simulink model "ProcessNetworkSimulation"  (R2015b)
settings: Solver=VariableStepAuto  StartTime=0.0  StopTime=1000.0  RelTol=1e-3
libraries: simulink x1, simeventslib x1
(part 20 of 21)

== system ProcessNetworkSimulation/Process_73/Process ==
  OUTQueue : FIFOQueue  Capacity=inf
  ProcessQueue : FIFOQueue  Capacity=Inf  StatAverageWait=on  StatAverageQueueLength=on
      settings: OutputPortMap=o2,o3
  ProcessServer : NServer  NumberOfServers=14  ServiceTimeFrom=Signal port t  StatNumberDeparted=on  StatUtilization=on
      settings: OutputPortMap=o0,o5
  ProcessTime : EventBasedRandomNumber  meanExp=0.05  minUnif=1  meanNorm=2  stdNorm=0.2  Seed=56201
  Routing : EventBasedRandomNumber  Distribution=Arbitrary discrete  valueVecDisc=[0,1,2,3,4,5,6,7,8,9,10,11,12,13,14,15,16,17,18,19,20,21,22,23,24,25,26,27,28,29,30,31,32,33,34,35,36,37,38,39,40,41,42,43,44]  probVecDisc=[0,0.032,0.0036,0.0071,0.0285,0.032,0.0071,0.032,0.0214,0.0249,0.0214,0.032,0.0036,0.032,0.0285,0.0249,0.0249,0.0249,0.0214,0.032,0.032,0.032,0.0249,0.0285,0.0249,0.0178,0.0214,0.032,0.032,0.0071,0.0071,0.032,0.0036,0.0356,0.0214,0.032,0.0249,0.0249,0.032,0.0107,0.0071,0.0214,0.0249,0.0285,0.0071]  Seed=59418
  read_ProcessTimer : ReadTimer  TimerTag=T_Process_73  StatAverageTimeElapsed=on
      settings: OutputPortMap=o3
  setRouting : SetAttribute  AttributeName=outputFlowNode  AttributeFrom=Signal port  EvaluatedAttributeValue={ []}
  start_ProcessTimer : StartTimer  TimerTag=T_Process_73  TimerStartedOption=Restart
  IN_Job : PMIOPort  Port=1  Side=Left
  OUT_Job : PMIOPort  Port=2  Side=Right
  wires:
  Routing/1 -> setRouting/1
  ProcessTime/1 -> ProcessServer/1
  connections:
  setRouting/LConn1 -- OUTQueue/RConn1
  IN_Job/RConn1 -- start_ProcessTimer/LConn1
  ProcessServer/RConn1 -- read_ProcessTimer/LConn1
  start_ProcessTimer/RConn1 -- ProcessQueue/LConn1
  ProcessQueue/RConn1 -- ProcessServer/LConn1
  read_ProcessTimer/RConn1 -- OUTQueue/LConn1
  OUT_Job/RConn1 -- setRouting/RConn1

== system ProcessNetworkSimulation/Process_74/Process ==
  OUTQueue : FIFOQueue  Capacity=inf
  ProcessQueue : FIFOQueue  Capacity=Inf  StatAverageWait=on  StatAverageQueueLength=on
      settings: OutputPortMap=o2,o3
  ProcessServer : NServer  NumberOfServers=8  ServiceTimeFrom=Signal port t  StatNumberDeparted=on  StatUtilization=on
      settings: OutputPortMap=o0,o5
  ProcessTime : EventBasedRandomNumber  meanExp=0.05  minUnif=1  meanNorm=2  stdNorm=0.2  Seed=62635
  Routing : EventBasedRandomNumber  Distribution=Arbitrary discrete  valueVecDisc=[0,1,2,3,4,5,6,7,8,9,10,11,12,13,14,15,16,17,18,19,20,21,22,23,24,25,26,27,28,29,30,31,32,33,34,35]  probVecDisc=[0,0.0511,0.0146,0.0146,0.0657,0.0219,0.0438,0.0365,0.0511,0.0365,0.0146,0.0146,0.0146,0.0657,0.0365,0.0146,0.0073,0.0146,0.0729,0.0365,0.0219,0.0219,0.0219,0.0146,0.0073,0.0146,0.0511,0.0365,0.0219,0.0146,0.0146,0.0073,0.0146,0.0438,0.0657,0]  Seed=316
  read_ProcessTimer : ReadTimer  TimerTag=T_Process_74  StatAverageTimeElapsed=on
      settings: OutputPortMap=o3
  setRouting : SetAttribute  AttributeName=outputFlowNode  AttributeFrom=Signal port  EvaluatedAttributeValue={ []}
  start_ProcessTimer : StartTimer  TimerTag=T_Process_74  TimerStartedOption=Restart
  IN_Job : PMIOPort  Port=1  Side=Left
  OUT_Job : PMIOPort  Port=2  Side=Right
  wires:
  Routing/1 -> setRouting/1
  ProcessTime/1 -> ProcessServer/1
  connections:
  setRouting/LConn1 -- OUTQueue/RConn1
  IN_Job/RConn1 -- start_ProcessTimer/LConn1
  ProcessServer/RConn1 -- read_ProcessTimer/LConn1
  start_ProcessTimer/RConn1 -- ProcessQueue/LConn1
  ProcessQueue/RConn1 -- ProcessServer/LConn1
  read_ProcessTimer/RConn1 -- OUTQueue/LConn1
  OUT_Job/RConn1 -- setRouting/RConn1

== system ProcessNetworkSimulation/Process_75/Process ==
  OUTQueue : FIFOQueue  Capacity=inf
  ProcessQueue : FIFOQueue  Capacity=Inf  StatAverageWait=on  StatAverageQueueLength=on
      settings: OutputPortMap=o2,o3
  ProcessServer : NServer  NumberOfServers=13  ServiceTimeFrom=Signal port t  StatNumberDeparted=on  StatUtilization=on
      settings: OutputPortMap=o0,o5
  ProcessTime : EventBasedRandomNumber  meanExp=0.05  minUnif=1  meanNorm=2  stdNorm=0.2  Seed=3533
  Routing : EventBasedRandomNumber  Distribution=Arbitrary discrete  valueVecDisc=[0,1,2,3,4,5,6,7,8,9,10,11,12,13,14,15,16,17,18,19,20,21,22,23,24,25,26,27,28,29,30,31,32,33,34,35,36,37,38,39,40,41,42,43,44,45,46,47,48,49,50]  probVecDisc=[0,0.0081,0.0242,0.0242,0.0242,0.004,0.0121,0.0363,0.0121,0.0081,0.0081,0.0363,0.0282,0.0397,0.0363,0.0081,0.0282,0.0081,0.0081,0.0323,0.0202,0.0363,0.0081,0.0202,0.0282,0.0081,0.0202,0.0081,0.004,0.0363,0.0121,0.0081,0.0242,0.0282,0.0363,0.0202,0.0242,0.0081,0.0282,0.0081,0.0363,0.0081,0.0282,0.0081,0.0242,0.0121,0.0242,0.0081,0.0403,0.0363,0]  Seed=6750
  read_ProcessTimer : ReadTimer  TimerTag=T_Process_75  StatAverageTimeElapsed=on
      settings: OutputPortMap=o3
  setRouting : SetAttribute  AttributeName=outputFlowNode  AttributeFrom=Signal port  EvaluatedAttributeValue={ []}
  start_ProcessTimer : StartTimer  TimerTag=T_Process_75  TimerStartedOption=Restart
  IN_Job : PMIOPort  Port=1  Side=Left
  OUT_Job : PMIOPort  Port=2  Side=Right
  wires:
  Routing/1 -> setRouting/1
  ProcessTime/1 -> ProcessServer/1
  connections:
  setRouting/LConn1 -- OUTQueue/RConn1
  IN_Job/RConn1 -- start_ProcessTimer/LConn1
  ProcessServer/RConn1 -- read_ProcessTimer/LConn1
  start_ProcessTimer/RConn1 -- ProcessQueue/LConn1
  ProcessQueue/RConn1 -- ProcessServer/LConn1
  read_ProcessTimer/RConn1 -- OUTQueue/LConn1
  OUT_Job/RConn1 -- setRouting/RConn1

== system ProcessNetworkSimulation/Process_76/Process ==
  OUTQueue : FIFOQueue  Capacity=inf
  ProcessQueue : FIFOQueue  Capacity=Inf  StatAverageWait=on  StatAverageQueueLength=on
      settings: OutputPortMap=o2,o3
  ProcessServer : NServer  NumberOfServers=13  ServiceTimeFrom=Signal port t  StatNumberDeparted=on  StatUtilization=on
      settings: OutputPortMap=o0,o5
  ProcessTime : EventBasedRandomNumber  meanExp=0.05  minUnif=1  meanNorm=2  stdNorm=0.2  Seed=9967
  Routing : EventBasedRandomNumber  Distribution=Arbitrary discrete  valueVecDisc=[0,1,2,3,4,5,6,7,8,9,10,11,12,13,14,15,16,17,18,19,20,21,22,23,24,25,26,27,28,29,30,31,32,33,34,35,36,37,38]  probVecDisc=[0,0.0433,0.0048,0.024,0.0096,0.024,0.0385,0.0096,0.0096,0.0288,0.024,0.0433,0.0337,0.0337,0.0433,0.0096,0.0096,0.0337,0.0337,0.0433,0.024,0.0144,0.0288,0.0481,0.0433,0.0096,0.0144,0.0433,0.0337,0.0096,0.024,0.0288,0.0288,0.024,0.0048,0.0385,0.0481,0.0337,0]  Seed=13184
  read_ProcessTimer : ReadTimer  TimerTag=T_Process_76  StatAverageTimeElapsed=on
      settings: OutputPortMap=o3
  setRouting : SetAttribute  AttributeName=outputFlowNode  AttributeFrom=Signal port  EvaluatedAttributeValue={ []}
  start_ProcessTimer : StartTimer  TimerTag=T_Process_76  TimerStartedOption=Restart
  IN_Job : PMIOPort  Port=1  Side=Left
  OUT_Job : PMIOPort  Port=2  Side=Right
  wires:
  Routing/1 -> setRouting/1
  ProcessTime/1 -> ProcessServer/1
  connections:
  setRouting/LConn1 -- OUTQueue/RConn1
  IN_Job/RConn1 -- start_ProcessTimer/LConn1
  ProcessServer/RConn1 -- read_ProcessTimer/LConn1
  start_ProcessTimer/RConn1 -- ProcessQueue/LConn1
  ProcessQueue/RConn1 -- ProcessServer/LConn1
  read_ProcessTimer/RConn1 -- OUTQueue/LConn1
  OUT_Job/RConn1 -- setRouting/RConn1

== system ProcessNetworkSimulation/Process_77/Process ==
  OUTQueue : FIFOQueue  Capacity=inf
  ProcessQueue : FIFOQueue  Capacity=Inf  StatAverageWait=on  StatAverageQueueLength=on
      settings: OutputPortMap=o2,o3
  ProcessServer : NServer  NumberOfServers=10  ServiceTimeFrom=Signal port t  StatNumberDeparted=on  StatUtilization=on
      settings: OutputPortMap=o0,o5
  ProcessTime : EventBasedRandomNumber  meanExp=0.05  minUnif=1  meanNorm=2  stdNorm=0.2  Seed=16401
  Routing : EventBasedRandomNumber  Distribution=Arbitrary discrete  valueVecDisc=[0,1,2,3,4,5,6,7,8,9,10,11,12,13,14,15,16,17,18,19,20,21,22,23,24,25,26,27,28,29,30,31,32,33,34,35,36,37,38]  probVecDisc=[0,0.0279,0.0112,0.0335,0.0112,0.0503,0.0335,0.0112,0.0112,0.0391,0.0168,0.0279,0.0112,0.0279,0.0335,0.0503,0.0112,0.0112,0.0335,0.0447,0.0112,0.0112,0.0503,0.0503,0.0391,0.0112,0.0556,0.0335,0.0279,0.0112,0.0112,0.0335,0.0279,0.0391,0.0391,0.0056,0.0168,0.0168,0.0112]  Seed=19618
  read_ProcessTimer : ReadTimer  TimerTag=T_Process_77  StatAverageTimeElapsed=on
      settings: OutputPortMap=o3
  setRouting : SetAttribute  AttributeName=outputFlowNode  AttributeFrom=Signal port  EvaluatedAttributeValue={ []}
  start_ProcessTimer : StartTimer  TimerTag=T_Process_77  TimerStartedOption=Restart
  IN_Job : PMIOPort  Port=1  Side=Left
  OUT_Job : PMIOPort  Port=2  Side=Right
  wires:
  Routing/1 -> setRouting/1
  ProcessTime/1 -> ProcessServer/1
  connections:
  setRouting/LConn1 -- OUTQueue/RConn1
  IN_Job/RConn1 -- start_ProcessTimer/LConn1
  ProcessServer/RConn1 -- read_ProcessTimer/LConn1
  start_ProcessTimer/RConn1 -- ProcessQueue/LConn1
  ProcessQueue/RConn1 -- ProcessServer/LConn1
  read_ProcessTimer/RConn1 -- OUTQueue/LConn1
  OUT_Job/RConn1 -- setRouting/RConn1

== system ProcessNetworkSimulation/Process_78/Process ==
  OUTQueue : FIFOQueue  Capacity=inf
  ProcessQueue : FIFOQueue  Capacity=Inf  StatAverageWait=on  StatAverageQueueLength=on
      settings: OutputPortMap=o2,o3
  ProcessServer : NServer  NumberOfServers=9  ServiceTimeFrom=Signal port t  StatNumberDeparted=on  StatUtilization=on
      settings: OutputPortMap=o0,o5
  ProcessTime : EventBasedRandomNumber  meanExp=0.05  minUnif=1  meanNorm=2  stdNorm=0.2  Seed=22835
  Routing : EventBasedRandomNumber  Distribution=Arbitrary discrete  valueVecDisc=[0,1,2,3,4,5,6,7,8,9,10,11,12,13,14,15,16,17,18,19,20,21,22,23,24,25,26,27,28,29,30]  probVecDisc=[0,0.0349,0.0116,0.0523,0.0291,0.0523,0.0349,0.0349,0.0116,0.0116,0.0584,0.0349,0.0581,0.0116,0.0116,0.0581,0.0407,0.0407,0.0523,0.0523,0.0116,0.0116,0.0291,0.0523,0.0407,0.0523,0.0291,0.0291,0.0407,0.0116,0]  Seed=26052
  read_ProcessTimer : ReadTimer  TimerTag=T_Process_78  StatAverageTimeElapsed=on
      settings: OutputPortMap=o3
  setRouting : SetAttribute  AttributeName=outputFlowNode  AttributeFrom=Signal port  EvaluatedAttributeValue={ []}
  start_ProcessTimer : StartTimer  TimerTag=T_Process_78  TimerStartedOption=Restart
  IN_Job : PMIOPort  Port=1  Side=Left
  OUT_Job : PMIOPort  Port=2  Side=Right
  wires:
  Routing/1 -> setRouting/1
  ProcessTime/1 -> ProcessServer/1
  connections:
  setRouting/LConn1 -- OUTQueue/RConn1
  IN_Job/RConn1 -- start_ProcessTimer/LConn1
  ProcessServer/RConn1 -- read_ProcessTimer/LConn1
  start_ProcessTimer/RConn1 -- ProcessQueue/LConn1
  ProcessQueue/RConn1 -- ProcessServer/LConn1
  read_ProcessTimer/RConn1 -- OUTQueue/LConn1
  OUT_Job/RConn1 -- setRouting/RConn1

== system ProcessNetworkSimulation/Process_79/Process ==
  OUTQueue : FIFOQueue  Capacity=inf
  ProcessQueue : FIFOQueue  Capacity=Inf  StatAverageWait=on  StatAverageQueueLength=on
      settings: OutputPortMap=o2,o3
  ProcessServer : NServer  NumberOfServers=13  ServiceTimeFrom=Signal port t  StatNumberDeparted=on  StatUtilization=on
      settings: OutputPortMap=o0,o5
  ProcessTime : EventBasedRandomNumber  meanExp=0.05  minUnif=1  meanNorm=2  stdNorm=0.2  Seed=29269
  Routing : EventBasedRandomNumber  Distribution=Arbitrary discrete  valueVecDisc=[0,1,2,3,4,5,6,7,8,9,10,11,12,13,14,15,16,17,18,19,20,21,22,23,24,25,26,27,28,29,30,31,32,33,34,35,36,37,38,39]  probVecDisc=[0,0.0136,0.0318,0.0273,0.0364,0.0091,0.0409,0.0318,0.0091,0.0409,0.0318,0.0227,0.0091,0.0318,0.0091,0.0273,0.0409,0.0091,0.0091,0.0136,0.0318,0.0409,0.0273,0.0091,0.0091,0.0455,0.0409,0.0273,0.0409,0.0409,0.0364,0.0455,0.0409,0.0409,0.0318,0.0091,0.0136,0.0091,0.0136,0]  Seed=32486
  read_ProcessTimer : ReadTimer  TimerTag=T_Process_79  StatAverageTimeElapsed=on
      settings: OutputPortMap=o3
  setRouting : SetAttribute  AttributeName=outputFlowNode  AttributeFrom=Signal port  EvaluatedAttributeValue={ []}
  start_ProcessTimer : StartTimer  TimerTag=T_Process_79  TimerStartedOption=Restart
  IN_Job : PMIOPort  Port=1  Side=Left
  OUT_Job : PMIOPort  Port=2  Side=Right
  wires:
  Routing/1 -> setRouting/1
  ProcessTime/1 -> ProcessServer/1
  connections:
  setRouting/LConn1 -- OUTQueue/RConn1
  IN_Job/RConn1 -- start_ProcessTimer/LConn1
  ProcessServer/RConn1 -- read_ProcessTimer/LConn1
  start_ProcessTimer/RConn1 -- ProcessQueue/LConn1
  ProcessQueue/RConn1 -- ProcessServer/LConn1
  read_ProcessTimer/RConn1 -- OUTQueue/LConn1
  OUT_Job/RConn1 -- setRouting/RConn1

== system ProcessNetworkSimulation/Process_8/Process ==
  OUTQueue : FIFOQueue  Capacity=inf
  ProcessQueue : FIFOQueue  Capacity=Inf  StatAverageWait=on  StatAverageQueueLength=on
      settings: OutputPortMap=o2,o3
  ProcessServer : NServer  NumberOfServers=11  ServiceTimeFrom=Signal port t  StatNumberDeparted=on  StatUtilization=on
      settings: OutputPortMap=o0,o5
  ProcessTime : EventBasedRandomNumber  meanExp=0.05  minUnif=1  meanNorm=2  stdNorm=0.2  Seed=35703
  Routing : EventBasedRandomNumber  Distribution=Arbitrary discrete  valueVecDisc=[0,1,2,3,4,5,6,7,8,9,10,11,12,13,14,15,16,17,18,19,20,21,22,23,24,25,26,27,28,29,30,31,32,33,34]  probVecDisc=[0,0.0448,0.0348,0.0448,0.0249,0.0398,0.01,0.0448,0.0492,0.01,0.0249,0.0348,0.005,0.0299,0.0448,0.0448,0.0348,0.0348,0.01,0.01,0.0249,0.0299,0.01,0.0398,0.01,0.0348,0.01,0.0348,0.01,0.0348,0.0348,0.0348,0.0448,0.0249,0.0448]  Seed=38920
  read_ProcessTimer : ReadTimer  TimerTag=T_Process_8  StatAverageTimeElapsed=on
      settings: OutputPortMap=o3
  setRouting : SetAttribute  AttributeName=outputFlowNode  AttributeFrom=Signal port  EvaluatedAttributeValue={ []}
  start_ProcessTimer : StartTimer  TimerTag=T_Process_8  TimerStartedOption=Restart
  IN_Job : PMIOPort  Port=1  Side=Left
  OUT_Job : PMIOPort  Port=2  Side=Right
  wires:
  Routing/1 -> setRouting/1
  ProcessTime/1 -> ProcessServer/1
  connections:
  setRouting/LConn1 -- OUTQueue/RConn1
  IN_Job/RConn1 -- start_ProcessTimer/LConn1
  ProcessServer/RConn1 -- read_ProcessTimer/LConn1
  start_ProcessTimer/RConn1 -- ProcessQueue/LConn1
  ProcessQueue/RConn1 -- ProcessServer/LConn1
  read_ProcessTimer/RConn1 -- OUTQueue/LConn1
  OUT_Job/RConn1 -- setRouting/RConn1

== system ProcessNetworkSimulation/Process_80/Process ==
  OUTQueue : FIFOQueue  Capacity=inf
  ProcessQueue : FIFOQueue  Capacity=Inf  StatAverageWait=on  StatAverageQueueLength=on
      settings: OutputPortMap=o2,o3
  ProcessServer : NServer  NumberOfServers=10  ServiceTimeFrom=Signal port t  StatNumberDeparted=on  StatUtilization=on
      settings: OutputPortMap=o0,o5
  ProcessTime : EventBasedRandomNumber  meanExp=0.05  minUnif=1  meanNorm=2  stdNorm=0.2  Seed=42137
  Routing : EventBasedRandomNumber  Distribution=Arbitrary discrete  valueVecDisc=[0,1,2,3,4,5,6,7,8,9,10,11,12,13,14,15,16,17,18,19,20,21,22,23,24,25,26,27,28,29,30,31,32,33,34,35,36,37,38,39,40,41]  probVecDisc=[0,0.0091,0.0136,0.0136,0.0457,0.0136,0.0409,0.0409,0.0409,0.0091,0.0227,0.0136,0.0318,0.0409,0.0091,0.0091,0.0318,0.0409,0.0409,0.0227,0.0318,0.0273,0.0136,0.0364,0.0273,0.0409,0.0136,0.0364,0.0091,0.0273,0.0364,0.0091,0.0409,0.0227,0.0091,0.0045,0.0227,0.0227,0.0273,0.0091,0.0409,0]  Seed=45354
  read_ProcessTimer : ReadTimer  TimerTag=T_Process_80  StatAverageTimeElapsed=on
      settings: OutputPortMap=o3
  setRouting : SetAttribute  AttributeName=outputFlowNode  AttributeFrom=Signal port  EvaluatedAttributeValue={ []}
  start_ProcessTimer : StartTimer  TimerTag=T_Process_80  TimerStartedOption=Restart
  IN_Job : PMIOPort  Port=1  Side=Left
  OUT_Job : PMIOPort  Port=2  Side=Right
  wires:
  Routing/1 -> setRouting/1
  ProcessTime/1 -> ProcessServer/1
  connections:
  setRouting/LConn1 -- OUTQueue/RConn1
  IN_Job/RConn1 -- start_ProcessTimer/LConn1
  ProcessServer/RConn1 -- read_ProcessTimer/LConn1
  start_ProcessTimer/RConn1 -- ProcessQueue/LConn1
  ProcessQueue/RConn1 -- ProcessServer/LConn1
  read_ProcessTimer/RConn1 -- OUTQueue/LConn1
  OUT_Job/RConn1 -- setRouting/RConn1

== system ProcessNetworkSimulation/Process_81/Process ==
  OUTQueue : FIFOQueue  Capacity=inf
  ProcessQueue : FIFOQueue  Capacity=Inf  StatAverageWait=on  StatAverageQueueLength=on
      settings: OutputPortMap=o2,o3
  ProcessServer : NServer  NumberOfServers=13  ServiceTimeFrom=Signal port t  StatNumberDeparted=on  StatUtilization=on
      settings: OutputPortMap=o0,o5
  ProcessTime : EventBasedRandomNumber  meanExp=0.05  minUnif=1  meanNorm=2  stdNorm=0.2  Seed=48571
  Routing : EventBasedRandomNumber  Distribution=Arbitrary discrete  valueVecDisc=[0,1,2,3,4,5,6,7,8,9,10,11,12,13,14,15,16,17,18,19,20,21,22,23,24,25,26,27,28,29,30,31,32,33,34,35,36,37,38]  probVecDisc=[0,0.0457,0.0411,0.0274,0.0137,0.032,0.0091,0.0411,0.032,0.0091,0.0228,0.0091,0.032,0.0457,0.032,0.0091,0.0091,0.0137,0.0274,0.0228,0.0091,0.0091,0.0411,0.0137,0.0274,0.0457,0.0228,0.0411,0.0137,0.0411,0.0411,0.032,0.0137,0.0365,0.0411,0.0137,0.0274,0.0274,0.0274]  Seed=51788
  read_ProcessTimer : ReadTimer  TimerTag=T_Process_81  StatAverageTimeElapsed=on
      settings: OutputPortMap=o3
  setRouting : SetAttribute  AttributeName=outputFlowNode  AttributeFrom=Signal port  EvaluatedAttributeValue={ []}
  start_ProcessTimer : StartTimer  TimerTag=T_Process_81  TimerStartedOption=Restart
  IN_Job : PMIOPort  Port=1  Side=Left
  OUT_Job : PMIOPort  Port=2  Side=Right
  wires:
  Routing/1 -> setRouting/1
  ProcessTime/1 -> ProcessServer/1
  connections:
  setRouting/LConn1 -- OUTQueue/RConn1
  IN_Job/RConn1 -- start_ProcessTimer/LConn1
  ProcessServer/RConn1 -- read_ProcessTimer/LConn1
  start_ProcessTimer/RConn1 -- ProcessQueue/LConn1
  ProcessQueue/RConn1 -- ProcessServer/LConn1
  read_ProcessTimer/RConn1 -- OUTQueue/LConn1
  OUT_Job/RConn1 -- setRouting/RConn1

== system ProcessNetworkSimulation/Process_82/Process ==
  OUTQueue : FIFOQueue  Capacity=inf
  ProcessQueue : FIFOQueue  Capacity=Inf  StatAverageWait=on  StatAverageQueueLength=on
      settings: OutputPortMap=o2,o3
  ProcessServer : NServer  NumberOfServers=14  ServiceTimeFrom=Signal port t  StatNumberDeparted=on  StatUtilization=on
      settings: OutputPortMap=o0,o5
  ProcessTime : EventBasedRandomNumber  meanExp=0.05  minUnif=1  meanNorm=2  stdNorm=0.2  Seed=55005
  Routing : EventBasedRandomNumber  Distribution=Arbitrary discrete  valueVecDisc=[0,1,2,3,4,5,6,7,8,9,10,11,12,13,14,15,16,17,18,19,20,21,22,23,24,25,26,27,28,29,30,31,32,33,34,35,36,37,38,39,40]  probVecDisc=[0,0.0248,0.0248,0.0372,0.0207,0.0289,0.0083,0.0248,0.0083,0.0331,0.0207,0.0248,0.0248,0.0372,0.0289,0.0372,0.0289,0.0372,0.0083,0.0372,0.0372,0.0207,0.0372,0.0083,0.0248,0.0041,0.0372,0.0372,0.0289,0.0372,0.0207,0.0372,0.041,0.0248,0.0248,0.0289,0.0124,0.0041,0.0331,0.0041,0]  Seed=58222
  read_ProcessTimer : ReadTimer  TimerTag=T_Process_82  StatAverageTimeElapsed=on
      settings: OutputPortMap=o3
  setRouting : SetAttribute  AttributeName=outputFlowNode  AttributeFrom=Signal port  EvaluatedAttributeValue={ []}
  start_ProcessTimer : StartTimer  TimerTag=T_Process_82  TimerStartedOption=Restart
  IN_Job : PMIOPort  Port=1  Side=Left
  OUT_Job : PMIOPort  Port=2  Side=Right
  wires:
  Routing/1 -> setRouting/1
  ProcessTime/1 -> ProcessServer/1
  connections:
  setRouting/LConn1 -- OUTQueue/RConn1
  IN_Job/RConn1 -- start_ProcessTimer/LConn1
  ProcessServer/RConn1 -- read_ProcessTimer/LConn1
  start_ProcessTimer/RConn1 -- ProcessQueue/LConn1
  ProcessQueue/RConn1 -- ProcessServer/LConn1
  read_ProcessTimer/RConn1 -- OUTQueue/LConn1
  OUT_Job/RConn1 -- setRouting/RConn1

== system ProcessNetworkSimulation/Process_83/Process ==
  OUTQueue : FIFOQueue  Capacity=inf
  ProcessQueue : FIFOQueue  Capacity=Inf  StatAverageWait=on  StatAverageQueueLength=on
      settings: OutputPortMap=o2,o3
  ProcessServer : NServer  NumberOfServers=10  ServiceTimeFrom=Signal port t  StatNumberDeparted=on  StatUtilization=on
      settings: OutputPortMap=o0,o5
  ProcessTime : EventBasedRandomNumber  meanExp=0.05  minUnif=1  meanNorm=2  stdNorm=0.2  Seed=61439
  Routing : EventBasedRandomNumber  Distribution=Arbitrary discrete  valueVecDisc=[0,1,2,3,4,5,6,7,8,9,10,11,12,13,14,15,16,17,18,19,20,21,22,23,24,25,26,27,28,29,30,31,32,33,34,35,36,37,38,39,40,41,42,43,44,45]  probVecDisc=[0,0.0415,0.0259,0.0104,0.0155,0.0466,0.0104,0.0104,0.0363,0.0104,0.0155,0.0104,0.0415,0.0311,0.0466,0.0466,0.0155,0.0104,0.0104,0.0363,0.0259,0.0104,0.0104,0.0363,0.0104,0.0155,0.0155,0.0311,0.0104,0.0513,0.0104,0.0259,0.0104,0.0104,0.0104,0.0259,0.0155,0.0104,0.0104,0.0415,0.0104,0.0363,0.0259,0.0259,0.0155,0.0259]  Seed=64656
  read_ProcessTimer : ReadTimer  TimerTag=T_Process_83  StatAverageTimeElapsed=on
      settings: OutputPortMap=o3
  setRouting : SetAttribute  AttributeName=outputFlowNode  AttributeFrom=Signal port  EvaluatedAttributeValue={ []}
  start_ProcessTimer : StartTimer  TimerTag=T_Process_83  TimerStartedOption=Restart
  IN_Job : PMIOPort  Port=1  Side=Left
  OUT_Job : PMIOPort  Port=2  Side=Right
  wires:
  Routing/1 -> setRouting/1
  ProcessTime/1 -> ProcessServer/1
  connections:
  setRouting/LConn1 -- OUTQueue/RConn1
  IN_Job/RConn1 -- start_ProcessTimer/LConn1
  ProcessServer/RConn1 -- read_ProcessTimer/LConn1
  start_ProcessTimer/RConn1 -- ProcessQueue/LConn1
  ProcessQueue/RConn1 -- ProcessServer/LConn1
  read_ProcessTimer/RConn1 -- OUTQueue/LConn1
  OUT_Job/RConn1 -- setRouting/RConn1

== system ProcessNetworkSimulation/Process_84/Process ==
  OUTQueue : FIFOQueue  Capacity=inf
  ProcessQueue : FIFOQueue  Capacity=Inf  StatAverageWait=on  StatAverageQueueLength=on
      settings: OutputPortMap=o2,o3
  ProcessServer : NServer  NumberOfServers=12  ServiceTimeFrom=Signal port t  StatNumberDeparted=on  StatUtilization=on
      settings: OutputPortMap=o0,o5
  ProcessTime : EventBasedRandomNumber  meanExp=0.05  minUnif=1  meanNorm=2  stdNorm=0.2  Seed=2337
  Routing : EventBasedRandomNumber  Distribution=Arbitrary discrete  valueVecDisc=[0,1,2,3,4,5,6,7,8,9,10,11,12,13,14,15,16,17,18,19,20,21,22,23,24,25,26,27,28,29,30,31,32,33,34,35,36,37,38,39,40]  probVecDisc=[0,0.0251,0.0101,0.0101,0.0452,0.0101,0.0101,0.0452,0.0402,0.0492,0.0101,0.0101,0.0302,0.0352,0.0452,0.0101,0.0251,0.0101,0.0101,0.0302,0.0101,0.0302,0.0101,0.0151,0.0352,0.0352,0.0251,0.0302,0.0503,0.0503,0.0302,0.0452,0.0402,0.0101,0.0101,0.0151,0.0101,0.0151,0.0302,0.0402,0]  Seed=5554
  read_ProcessTimer : ReadTimer  TimerTag=T_Process_84  StatAverageTimeElapsed=on
      settings: OutputPortMap=o3
  setRouting : SetAttribute  AttributeName=outputFlowNode  AttributeFrom=Signal port  EvaluatedAttributeValue={ []}
  start_ProcessTimer : StartTimer  TimerTag=T_Process_84  TimerStartedOption=Restart
  IN_Job : PMIOPort  Port=1  Side=Left
  OUT_Job : PMIOPort  Port=2  Side=Right
  wires:
  Routing/1 -> setRouting/1
  ProcessTime/1 -> ProcessServer/1
  connections:
  setRouting/LConn1 -- OUTQueue/RConn1
  IN_Job/RConn1 -- start_ProcessTimer/LConn1
  ProcessServer/RConn1 -- read_ProcessTimer/LConn1
  start_ProcessTimer/RConn1 -- ProcessQueue/LConn1
  ProcessQueue/RConn1 -- ProcessServer/LConn1
  read_ProcessTimer/RConn1 -- OUTQueue/LConn1
  OUT_Job/RConn1 -- setRouting/RConn1

== system ProcessNetworkSimulation/Process_85/Process ==
  OUTQueue : FIFOQueue  Capacity=inf
  ProcessQueue : FIFOQueue  Capacity=Inf  StatAverageWait=on  StatAverageQueueLength=on
      settings: OutputPortMap=o2,o3
  ProcessServer : NServer  NumberOfServers=13  ServiceTimeFrom=Signal port t  StatNumberDeparted=on  StatUtilization=on
      settings: OutputPortMap=o0,o5
  ProcessTime : EventBasedRandomNumber  meanExp=0.05  minUnif=1  meanNorm=2  stdNorm=0.2  Seed=8771
  Routing : EventBasedRandomNumber  Distribution=Arbitrary discrete  valueVecDisc=[0,1,2,3,4,5,6,7,8,9,10,11,12,13,14,15,16,17,18,19,20,21,22,23,24,25,26,27,28,29,30,31,32,33,34,35,36,37,38]  probVecDisc=[0,0.0348,0.01,0.01,0.0249,0.0299,0.01,0.0249,0.0448,0.0249,0.0249,0.0448,0.0448,0.01,0.0398,0.01,0.0249,0.0489,0.0348,0.0299,0.0249,0.0398,0.0249,0.0448,0.0348,0.0398,0.01,0.01,0.0299,0.0149,0.0149,0.0448,0.0348,0.01,0.0448,0.01,0.01,0.0299,0]  Seed=11988
  read_ProcessTimer : ReadTimer  TimerTag=T_Process_85  StatAverageTimeElapsed=on
      settings: OutputPortMap=o3
  setRouting : SetAttribute  AttributeName=outputFlowNode  AttributeFrom=Signal port  EvaluatedAttributeValue={ []}
  start_ProcessTimer : StartTimer  TimerTag=T_Process_85  TimerStartedOption=Restart
  IN_Job : PMIOPort  Port=1  Side=Left
  OUT_Job : PMIOPort  Port=2  Side=Right
  wires:
  Routing/1 -> setRouting/1
  ProcessTime/1 -> ProcessServer/1
  connections:
  setRouting/LConn1 -- OUTQueue/RConn1
  IN_Job/RConn1 -- start_ProcessTimer/LConn1
  ProcessServer/RConn1 -- read_ProcessTimer/LConn1
  start_ProcessTimer/RConn1 -- ProcessQueue/LConn1
  ProcessQueue/RConn1 -- ProcessServer/LConn1
  read_ProcessTimer/RConn1 -- OUTQueue/LConn1
  OUT_Job/RConn1 -- setRouting/RConn1

== system ProcessNetworkSimulation/Process_86/Process ==
  OUTQueue : FIFOQueue  Capacity=inf
  ProcessQueue : FIFOQueue  Capacity=Inf  StatAverageWait=on  StatAverageQueueLength=on
      settings: OutputPortMap=o2,o3
  ProcessServer : NServer  NumberOfServers=10  ServiceTimeFrom=Signal port t  StatNumberDeparted=on  StatUtilization=on
      settings: OutputPortMap=o0,o5
  ProcessTime : EventBasedRandomNumber  meanExp=0.05  minUnif=1  meanNorm=2  stdNorm=0.2  Seed=15205
  Routing : EventBasedRandomNumber  Distribution=Arbitrary discrete  valueVecDisc=[0,1,2,3,4,5,6,7,8,9,10,11,12,13,14,15,16,17,18,19,20,21,22,23,24,25,26,27,28,29,30,31,32,33,34,35,36,37,38]  probVecDisc=[0,0.0323,0.0269,0.0484,0.0376,0.0376,0.0054,0.0484,0.0323,0.0484,0.0533,0.0269,0.0108,0.0161,0.0376,0.0269,0.0323,0.0376,0.0108,0.0108,0.0323,0.0161,0.0161,0.0108,0.0323,0.0376,0.0108,0.0269,0.0108,0.0161,0.0323,0.0161,0.0108,0.0323,0.043,0.0108,0.0269,0.0376,0]  Seed=18422
  read_ProcessTimer : ReadTimer  TimerTag=T_Process_86  StatAverageTimeElapsed=on
      settings: OutputPortMap=o3
  setRouting : SetAttribute  AttributeName=outputFlowNode  AttributeFrom=Signal port  EvaluatedAttributeValue={ []}
  start_ProcessTimer : StartTimer  TimerTag=T_Process_86  TimerStartedOption=Restart
  IN_Job : PMIOPort  Port=1  Side=Left
  OUT_Job : PMIOPort  Port=2  Side=Right
  wires:
  Routing/1 -> setRouting/1
  ProcessTime/1 -> ProcessServer/1
  connections:
  setRouting/LConn1 -- OUTQueue/RConn1
  IN_Job/RConn1 -- start_ProcessTimer/LConn1
  ProcessServer/RConn1 -- read_ProcessTimer/LConn1
  start_ProcessTimer/RConn1 -- ProcessQueue/LConn1
  ProcessQueue/RConn1 -- ProcessServer/LConn1
  read_ProcessTimer/RConn1 -- OUTQueue/LConn1
  OUT_Job/RConn1 -- setRouting/RConn1

== system ProcessNetworkSimulation/Process_87/Process ==
  OUTQueue : FIFOQueue  Capacity=inf
  ProcessQueue : FIFOQueue  Capacity=Inf  StatAverageWait=on  StatAverageQueueLength=on
      settings: OutputPortMap=o2,o3
  ProcessServer : NServer  NumberOfServers=11  ServiceTimeFrom=Signal port t  StatNumberDeparted=on  StatUtilization=on
      settings: OutputPortMap=o0,o5
  ProcessTime : EventBasedRandomNumber  meanExp=0.05  minUnif=1  meanNorm=2  stdNorm=0.2  Seed=21639
  Routing : EventBasedRandomNumber  Distribution=Arbitrary discrete  valueVecDisc=[0,1,2,3,4,5,6,7,8,9,10,11,12,13,14,15,16,17,18,19,20,21,22,23,24,25,26,27,28,29,30,31,32,33,34,35,36,37]  probVecDisc=[0,0.01,0.01,0.01,0.03,0.05,0.05,0.005,0.01,0.025,0.045,0.005,0.01,0.045,0.01,0.035,0.03,0.045,0.01,0.025,0.04,0.045,0.025,0.01,0.03,0.035,0.015,0.045,0.045,0.035,0.05,0.01,0.035,0.035,0.015,0.01,0.01,0.05]  Seed=24856
  read_ProcessTimer : ReadTimer  TimerTag=T_Process_87  StatAverageTimeElapsed=on
      settings: OutputPortMap=o3
  setRouting : SetAttribute  AttributeName=outputFlowNode  AttributeFrom=Signal port  EvaluatedAttributeValue={ []}
  start_ProcessTimer : StartTimer  TimerTag=T_Process_87  TimerStartedOption=Restart
  IN_Job : PMIOPort  Port=1  Side=Left
  OUT_Job : PMIOPort  Port=2  Side=Right
  wires:
  Routing/1 -> setRouting/1
  ProcessTime/1 -> ProcessServer/1
  connections:
  setRouting/LConn1 -- OUTQueue/RConn1
  IN_Job/RConn1 -- start_ProcessTimer/LConn1
  ProcessServer/RConn1 -- read_ProcessTimer/LConn1
  start_ProcessTimer/RConn1 -- ProcessQueue/LConn1
  ProcessQueue/RConn1 -- ProcessServer/LConn1
  read_ProcessTimer/RConn1 -- OUTQueue/LConn1
  OUT_Job/RConn1 -- setRouting/RConn1

== system ProcessNetworkSimulation/Process_88/Process ==
  OUTQueue : FIFOQueue  Capacity=inf
  ProcessQueue : FIFOQueue  Capacity=Inf  StatAverageWait=on  StatAverageQueueLength=on
      settings: OutputPortMap=o2,o3
  ProcessServer : NServer  NumberOfServers=10  ServiceTimeFrom=Signal port t  StatNumberDeparted=on  StatUtilization=on
      settings: OutputPortMap=o0,o5
  ProcessTime : EventBasedRandomNumber  meanExp=0.05  minUnif=1  meanNorm=2  stdNorm=0.2  Seed=28073
  Routing : EventBasedRandomNumber  Distribution=Arbitrary discrete  valueVecDisc=[0,1,2,3,4,5,6,7,8,9,10,11,12,13,14,15,16,17,18,19,20,21,22,23,24,25,26,27,28,29,30]  probVecDisc=[0,0.0476,0.0476,0.0532,0.0119,0.0119,0.0357,0.0119,0.0417,0.0417,0.0119,0.0357,0.0298,0.0298,0.0119,0.0536,0.0536,0.0357,0.0536,0.0298,0.0536,0.0119,0.0298,0.0536,0.0179,0.0417,0.0298,0.0476,0.0536,0.0119,0]  Seed=31290
  read_ProcessTimer : ReadTimer  TimerTag=T_Process_88  StatAverageTimeElapsed=on
      settings: OutputPortMap=o3
  setRouting : SetAttribute  AttributeName=outputFlowNode  AttributeFrom=Signal port  EvaluatedAttributeValue={ []}
  start_ProcessTimer : StartTimer  TimerTag=T_Process_88  TimerStartedOption=Restart
  IN_Job : PMIOPort  Port=1  Side=Left
  OUT_Job : PMIOPort  Port=2  Side=Right
  wires:
  Routing/1 -> setRouting/1
  ProcessTime/1 -> ProcessServer/1
  connections:
  setRouting/LConn1 -- OUTQueue/RConn1
  IN_Job/RConn1 -- start_ProcessTimer/LConn1
  ProcessServer/RConn1 -- read_ProcessTimer/LConn1
  start_ProcessTimer/RConn1 -- ProcessQueue/LConn1
  ProcessQueue/RConn1 -- ProcessServer/LConn1
  read_ProcessTimer/RConn1 -- OUTQueue/LConn1
  OUT_Job/RConn1 -- setRouting/RConn1

== system ProcessNetworkSimulation/Process_89/Process ==
  OUTQueue : FIFOQueue  Capacity=inf
  ProcessQueue : FIFOQueue  Capacity=Inf  StatAverageWait=on  StatAverageQueueLength=on
      settings: OutputPortMap=o2,o3
  ProcessServer : NServer  NumberOfServers=15  ServiceTimeFrom=Signal port t  StatNumberDeparted=on  StatUtilization=on
      settings: OutputPortMap=o0,o5
  ProcessTime : EventBasedRandomNumber  meanExp=0.05  minUnif=1  meanNorm=2  stdNorm=0.2  Seed=34507
  Routing : EventBasedRandomNumber  Distribution=Arbitrary discrete  valueVecDisc=[0,1,2,3,4,5,6,7,8,9,10,11,12,13,14,15,16,17,18,19,20,21,22,23,24,25,26,27,28,29,30,31,32,33,34,35,36,37,38,39,40]  probVecDisc=[0,0.0078,0.0352,0.0195,0.0313,0.0273,0.0273,0.0352,0.0313,0.0117,0.0039,0.0234,0.0273,0.0352,0.0273,0.0273,0.0273,0.0117,0.0352,0.0392,0.0195,0.0078,0.0352,0.0352,0.0078,0.0273,0.0078,0.0234,0.0078,0.0352,0.0352,0.0273,0.0313,0.0078,0.0273,0.0313,0.0234,0.0352,0.0273,0.0391,0.0234]  Seed=37724
  read_ProcessTimer : ReadTimer  TimerTag=T_Process_89  StatAverageTimeElapsed=on
      settings: OutputPortMap=o3
  setRouting : SetAttribute  AttributeName=outputFlowNode  AttributeFrom=Signal port  EvaluatedAttributeValue={ []}
  start_ProcessTimer : StartTimer  TimerTag=T_Process_89  TimerStartedOption=Restart
  IN_Job : PMIOPort  Port=1  Side=Left
  OUT_Job : PMIOPort  Port=2  Side=Right
  wires:
  Routing/1 -> setRouting/1
  ProcessTime/1 -> ProcessServer/1
  connections:
  setRouting/LConn1 -- OUTQueue/RConn1
  IN_Job/RConn1 -- start_ProcessTimer/LConn1
  ProcessServer/RConn1 -- read_ProcessTimer/LConn1
  start_ProcessTimer/RConn1 -- ProcessQueue/LConn1
  ProcessQueue/RConn1 -- ProcessServer/LConn1
  read_ProcessTimer/RConn1 -- OUTQueue/LConn1
  OUT_Job/RConn1 -- setRouting/RConn1

== system ProcessNetworkSimulation/Process_9/Process ==
  OUTQueue : FIFOQueue  Capacity=inf
  ProcessQueue : FIFOQueue  Capacity=Inf  StatAverageWait=on  StatAverageQueueLength=on
      settings: OutputPortMap=o2,o3
  ProcessServer : NServer  NumberOfServers=13  ServiceTimeFrom=Signal port t  StatNumberDeparted=on  StatUtilization=on
      settings: OutputPortMap=o0,o5
  ProcessTime : EventBasedRandomNumber  meanExp=0.05  minUnif=1  meanNorm=2  stdNorm=0.2  Seed=40941
  Routing : EventBasedRandomNumber  Distribution=Arbitrary discrete  valueVecDisc=[0,1,2,3,4,5,6,7,8,9,10,11,12,13,14,15,16,17,18,19,20,21,22,23,24,25,26,27,28,29,30,31,32,33,34,35,36,37,38,39,40,41,42,43]  probVecDisc=[0,0.0293,0.0126,0.041,0.0377,0.0293,0.0084,0.0209,0.0084,0.0377,0.0251,0.0084,0.0335,0.0377,0.0209,0.0084,0.0377,0.0084,0.0084,0.0293,0.0042,0.0377,0.0251,0.0084,0.0209,0.0377,0.0126,0.0251,0.0209,0.0293,0.0335,0.0209,0.0251,0.0293,0.0377,0.0084,0.0251,0.0084,0.0084,0.0251,0.0293,0.0377,0.0377,0.0084]  Seed=44158
  read_ProcessTimer : ReadTimer  TimerTag=T_Process_9  StatAverageTimeElapsed=on
      settings: OutputPortMap=o3
  setRouting : SetAttribute  AttributeName=outputFlowNode  AttributeFrom=Signal port  EvaluatedAttributeValue={ []}
  start_ProcessTimer : StartTimer  TimerTag=T_Process_9  TimerStartedOption=Restart
  IN_Job : PMIOPort  Port=1  Side=Left
  OUT_Job : PMIOPort  Port=2  Side=Right
  wires:
  Routing/1 -> setRouting/1
  ProcessTime/1 -> ProcessServer/1
  connections:
  setRouting/LConn1 -- OUTQueue/RConn1
  IN_Job/RConn1 -- start_ProcessTimer/LConn1
  ProcessServer/RConn1 -- read_ProcessTimer/LConn1
  start_ProcessTimer/RConn1 -- ProcessQueue/LConn1
  ProcessQueue/RConn1 -- ProcessServer/LConn1
  read_ProcessTimer/RConn1 -- OUTQueue/LConn1
  OUT_Job/RConn1 -- setRouting/RConn1

== system ProcessNetworkSimulation/Process_90/Process ==
  OUTQueue : FIFOQueue  Capacity=inf
  ProcessQueue : FIFOQueue  Capacity=Inf  StatAverageWait=on  StatAverageQueueLength=on
      settings: OutputPortMap=o2,o3
  ProcessServer : NServer  NumberOfServers=14  ServiceTimeFrom=Signal port t  StatNumberDeparted=on  StatUtilization=on
      settings: OutputPortMap=o0,o5
  ProcessTime : EventBasedRandomNumber  meanExp=0.05  minUnif=1  meanNorm=2  stdNorm=0.2  Seed=47375
  Routing : EventBasedRandomNumber  Distribution=Arbitrary discrete  valueVecDisc=[0,1,2,3,4,5,6,7,8,9,10,11,12,13,14,15,16,17,18,19,20,21,22,23,24,25,26,27,28,29,30,31,32,33,34,35,36,37,38,39,40]  probVecDisc=[0,0.0396,0.0088,0.0308,0.0449,0.0396,0.0264,0.022,0.0352,0.0088,0.0088,0.0132,0.0441,0.0396,0.0132,0.0088,0.0396,0.022,0.022,0.0396,0.022,0.0264,0.0264,0.0132,0.0132,0.0264,0.0352,0.0441,0.0044,0.0088,0.0088,0.0441,0.0088,0.0396,0.0264,0.0308,0.0396,0.0088,0.0352,0.0308,0]  Seed=50592
  read_ProcessTimer : ReadTimer  TimerTag=T_Process_90  StatAverageTimeElapsed=on
      settings: OutputPortMap=o3
  setRouting : SetAttribute  AttributeName=outputFlowNode  AttributeFrom=Signal port  EvaluatedAttributeValue={ []}
  start_ProcessTimer : StartTimer  TimerTag=T_Process_90  TimerStartedOption=Restart
  IN_Job : PMIOPort  Port=1  Side=Left
  OUT_Job : PMIOPort  Port=2  Side=Right
  wires:
  Routing/1 -> setRouting/1
  ProcessTime/1 -> ProcessServer/1
  connections:
  setRouting/LConn1 -- OUTQueue/RConn1
  IN_Job/RConn1 -- start_ProcessTimer/LConn1
  ProcessServer/RConn1 -- read_ProcessTimer/LConn1
  start_ProcessTimer/RConn1 -- ProcessQueue/LConn1
  ProcessQueue/RConn1 -- ProcessServer/LConn1
  read_ProcessTimer/RConn1 -- OUTQueue/LConn1
  OUT_Job/RConn1 -- setRouting/RConn1

== system ProcessNetworkSimulation/Process_91/Process ==
  OUTQueue : FIFOQueue  Capacity=inf
  ProcessQueue : FIFOQueue  Capacity=Inf  StatAverageWait=on  StatAverageQueueLength=on
      settings: OutputPortMap=o2,o3
  ProcessServer : NServer  NumberOfServers=13  ServiceTimeFrom=Signal port t  StatNumberDeparted=on  StatUtilization=on
      settings: OutputPortMap=o0,o5
  ProcessTime : EventBasedRandomNumber  meanExp=0.05  minUnif=1  meanNorm=2  stdNorm=0.2  Seed=53809
  Routing : EventBasedRandomNumber  Distribution=Arbitrary discrete  valueVecDisc=[0,1,2,3,4,5,6,7,8,9,10,11,12,13,14,15,16,17,18,19,20,21,22,23,24,25,26,27,28,29,30,31,32,33,34,35,36,37,38,39,40,41,42,43,44,45]  probVecDisc=[0,0.004,0.0361,0.012,0.012,0.0361,0.008,0.0241,0.0281,0.0281,0.008,0.004,0.004,0.0361,0.0321,0.012,0.008,0.0281,0.0281,0.0412,0.0281,0.0241,0.012,0.012,0.0241,0.004,0.0321,0.008,0.0201,0.0361,0.008,0.0361,0.0281,0.0402,0.0361,0.0281,0.008,0.0402,0.0361,0.012,0.008,0.0201,0.008,0.0361,0.0361,0.0281]  Seed=57026
  read_ProcessTimer : ReadTimer  TimerTag=T_Process_91  StatAverageTimeElapsed=on
      settings: OutputPortMap=o3
  setRouting : SetAttribute  AttributeName=outputFlowNode  AttributeFrom=Signal port  EvaluatedAttributeValue={ []}
  start_ProcessTimer : StartTimer  TimerTag=T_Process_91  TimerStartedOption=Restart
  IN_Job : PMIOPort  Port=1  Side=Left
  OUT_Job : PMIOPort  Port=2  Side=Right
  wires:
  Routing/1 -> setRouting/1
  ProcessTime/1 -> ProcessServer/1
  connections:
  setRouting/LConn1 -- OUTQueue/RConn1
  IN_Job/RConn1 -- start_ProcessTimer/LConn1
  ProcessServer/RConn1 -- read_ProcessTimer/LConn1
  start_ProcessTimer/RConn1 -- ProcessQueue/LConn1
  ProcessQueue/RConn1 -- ProcessServer/LConn1
  read_ProcessTimer/RConn1 -- OUTQueue/LConn1
  OUT_Job/RConn1 -- setRouting/RConn1

== system ProcessNetworkSimulation/Process_92/Process ==
  OUTQueue : FIFOQueue  Capacity=inf
  ProcessQueue : FIFOQueue  Capacity=Inf  StatAverageWait=on  StatAverageQueueLength=on
      settings: OutputPortMap=o2,o3
  ProcessServer : NServer  NumberOfServers=11  ServiceTimeFrom=Signal port t  StatNumberDeparted=on  StatUtilization=on
      settings: OutputPortMap=o0,o5
  ProcessTime : EventBasedRandomNumber  meanExp=0.05  minUnif=1  meanNorm=2  stdNorm=0.2  Seed=60243
  Routing : EventBasedRandomNumber  Distribution=Arbitrary discrete  valueVecDisc=[0,1,2,3,4,5,6,7,8,9,10,11,12,13,14,15,16,17,18,19,20,21,22,23,24,25,26,27,28,29,30,31,32,33,34,35,36]  probVecDisc=[0,0.033,0.0275,0.044,0.011,0.0165,0.0385,0.011,0.011,0.0275,0.0385,0.0385,0.011,0.0385,0.033,0.033,0.0165,0.011,0.0165,0.0385,0.0275,0.033,0.0485,0.011,0.0165,0.0275,0.0495,0.011,0.0165,0.0165,0.0495,0.0275,0.0495,0.011,0.0495,0.0275,0.033]  Seed=63460
  read_ProcessTimer : ReadTimer  TimerTag=T_Process_92  StatAverageTimeElapsed=on
      settings: OutputPortMap=o3
  setRouting : SetAttribute  AttributeName=outputFlowNode  AttributeFrom=Signal port  EvaluatedAttributeValue={ []}
  start_ProcessTimer : StartTimer  TimerTag=T_Process_92  TimerStartedOption=Restart
  IN_Job : PMIOPort  Port=1  Side=Left
  OUT_Job : PMIOPort  Port=2  Side=Right
  wires:
  Routing/1 -> setRouting/1
  ProcessTime/1 -> ProcessServer/1
  connections:
  setRouting/LConn1 -- OUTQueue/RConn1
  IN_Job/RConn1 -- start_ProcessTimer/LConn1
  ProcessServer/RConn1 -- read_ProcessTimer/LConn1
  start_ProcessTimer/RConn1 -- ProcessQueue/LConn1
  ProcessQueue/RConn1 -- ProcessServer/LConn1
  read_ProcessTimer/RConn1 -- OUTQueue/LConn1
  OUT_Job/RConn1 -- setRouting/RConn1

== system ProcessNetworkSimulation/Process_93/Process ==
  OUTQueue : FIFOQueue  Capacity=inf
  ProcessQueue : FIFOQueue  Capacity=Inf  StatAverageWait=on  StatAverageQueueLength=on
      settings: OutputPortMap=o2,o3
  ProcessServer : NServer  NumberOfServers=11  ServiceTimeFrom=Signal port t  StatNumberDeparted=on  StatUtilization=on
      settings: OutputPortMap=o0,o5
  ProcessTime : EventBasedRandomNumber  meanExp=0.05  minUnif=1  meanNorm=2  stdNorm=0.2  Seed=1141
  Routing : EventBasedRandomNumber  Distribution=Arbitrary discrete  valueVecDisc=[0,1,2,3,4,5,6,7,8,9,10,11,12,13,14,15,16,17,18,19,20,21,22,23,24,25,26,27,28,29,30,31,32,33,34,35,36,37,38,39,40]  probVecDisc=[0,0.0449,0.0102,0.0457,0.0305,0.0305,0.0355,0.0102,0.0152,0.0102,0.0355,0.0152,0.0305,0.0254,0.0305,0.0051,0.0254,0.0254,0.0254,0.0305,0.0254,0.0406,0.0152,0.0355,0.0355,0.0305,0.0152,0.0305,0.0102,0.0102,0.0102,0.0051,0.0305,0.0102,0.0457,0.0102,0.0102,0.0305,0.0305,0.0457,0.0406]  Seed=4358
  read_ProcessTimer : ReadTimer  TimerTag=T_Process_93  StatAverageTimeElapsed=on
      settings: OutputPortMap=o3
  setRouting : SetAttribute  AttributeName=outputFlowNode  AttributeFrom=Signal port  EvaluatedAttributeValue={ []}
  start_ProcessTimer : StartTimer  TimerTag=T_Process_93  TimerStartedOption=Restart
  IN_Job : PMIOPort  Port=1  Side=Left
  OUT_Job : PMIOPort  Port=2  Side=Right
  wires:
  Routing/1 -> setRouting/1
  ProcessTime/1 -> ProcessServer/1
  connections:
  setRouting/LConn1 -- OUTQueue/RConn1
  IN_Job/RConn1 -- start_ProcessTimer/LConn1
  ProcessServer/RConn1 -- read_ProcessTimer/LConn1
  start_ProcessTimer/RConn1 -- ProcessQueue/LConn1
  ProcessQueue/RConn1 -- ProcessServer/LConn1
  read_ProcessTimer/RConn1 -- OUTQueue/LConn1
  OUT_Job/RConn1 -- setRouting/RConn1

== system ProcessNetworkSimulation/Process_94/Process ==
  OUTQueue : FIFOQueue  Capacity=inf
  ProcessQueue : FIFOQueue  Capacity=Inf  StatAverageWait=on  StatAverageQueueLength=on
      settings: OutputPortMap=o2,o3
  ProcessServer : NServer  NumberOfServers=12  ServiceTimeFrom=Signal port t  StatNumberDeparted=on  StatUtilization=on
      settings: OutputPortMap=o0,o5
  ProcessTime : EventBasedRandomNumber  meanExp=0.05  minUnif=1  meanNorm=2  stdNorm=0.2  Seed=7575
  Routing : EventBasedRandomNumber  Distribution=Arbitrary discrete  valueVecDisc=[0,1,2,3,4,5,6,7,8,9,10,11,12,13,14,15,16,17,18,19,20,21,22,23,24,25,26,27,28,29,30,31,32,33,34,35,36,37,38,39,40,41,42,43,44]  probVecDisc=[0,0.0126,0.0126,0.0293,0.0084,0.0126,0.0293,0.0251,0.0042,0.0209,0.0293,0.0377,0.0293,0.0209,0.0251,0.0126,0.0209,0.0293,0.0293,0.0293,0.0377,0.0335,0.0251,0.0377,0.0126,0.0377,0.0084,0.0084,0.0209,0.0084,0.0084,0.0084,0.0251,0.0251,0.0251,0.0126,0.0209,0.0411,0.0377,0.0084,0.0209,0.0293,0.0251,0.0335,0.0293]  Seed=10792
  read_ProcessTimer : ReadTimer  TimerTag=T_Process_94  StatAverageTimeElapsed=on
      settings: OutputPortMap=o3
  setRouting : SetAttribute  AttributeName=outputFlowNode  AttributeFrom=Signal port  EvaluatedAttributeValue={ []}
  start_ProcessTimer : StartTimer  TimerTag=T_Process_94  TimerStartedOption=Restart
  IN_Job : PMIOPort  Port=1  Side=Left
  OUT_Job : PMIOPort  Port=2  Side=Right
  wires:
  Routing/1 -> setRouting/1
  ProcessTime/1 -> ProcessServer/1
  connections:
  setRouting/LConn1 -- OUTQueue/RConn1
  IN_Job/RConn1 -- start_ProcessTimer/LConn1
  ProcessServer/RConn1 -- read_ProcessTimer/LConn1
  start_ProcessTimer/RConn1 -- ProcessQueue/LConn1
  ProcessQueue/RConn1 -- ProcessServer/LConn1
  read_ProcessTimer/RConn1 -- OUTQueue/LConn1
  OUT_Job/RConn1 -- setRouting/RConn1

== system ProcessNetworkSimulation/Process_95/Process ==
  OUTQueue : FIFOQueue  Capacity=inf
  ProcessQueue : FIFOQueue  Capacity=Inf  StatAverageWait=on  StatAverageQueueLength=on
      settings: OutputPortMap=o2,o3
  ProcessServer : NServer  NumberOfServers=8  ServiceTimeFrom=Signal port t  StatNumberDeparted=on  StatUtilization=on
      settings: OutputPortMap=o0,o5
  ProcessTime : EventBasedRandomNumber  meanExp=0.05  minUnif=1  meanNorm=2  stdNorm=0.2  Seed=14009
  Routing : EventBasedRandomNumber  Distribution=Arbitrary discrete  valueVecDisc=[0,1,2,3,4,5,6,7,8,9,10,11,12,13,14,15,16,17,18,19,20,21,22,23,24,25,26,27,28,29,30,31,32,33,34,35]  probVecDisc=[0,0.006,0.055,0.012,0.0422,0.0482,0.012,0.0542,0.012,0.0542,0.012,0.0181,0.012,0.0422,0.0542,0.0181,0.0361,0.0181,0.0542,0.0301,0.012,0.0542,0.012,0.0482,0.0542,0.0301,0.0361,0.012,0.012,0.0361,0.0301,0.012,0.0361,0.012,0.012,0]  Seed=17226
  read_ProcessTimer : ReadTimer  TimerTag=T_Process_95  StatAverageTimeElapsed=on
      settings: OutputPortMap=o3
  setRouting : SetAttribute  AttributeName=outputFlowNode  AttributeFrom=Signal port  EvaluatedAttributeValue={ []}
  start_ProcessTimer : StartTimer  TimerTag=T_Process_95  TimerStartedOption=Restart
  IN_Job : PMIOPort  Port=1  Side=Left
  OUT_Job : PMIOPort  Port=2  Side=Right
  wires:
  Routing/1 -> setRouting/1
  ProcessTime/1 -> ProcessServer/1
  connections:
  setRouting/LConn1 -- OUTQueue/RConn1
  IN_Job/RConn1 -- start_ProcessTimer/LConn1
  ProcessServer/RConn1 -- read_ProcessTimer/LConn1
  start_ProcessTimer/RConn1 -- ProcessQueue/LConn1
  ProcessQueue/RConn1 -- ProcessServer/LConn1
  read_ProcessTimer/RConn1 -- OUTQueue/LConn1
  OUT_Job/RConn1 -- setRouting/RConn1

== system ProcessNetworkSimulation/Process_96/Process ==
  OUTQueue : FIFOQueue  Capacity=inf
  ProcessQueue : FIFOQueue  Capacity=Inf  StatAverageWait=on  StatAverageQueueLength=on
      settings: OutputPortMap=o2,o3
  ProcessServer : NServer  NumberOfServers=15  ServiceTimeFrom=Signal port t  StatNumberDeparted=on  StatUtilization=on
      settings: OutputPortMap=o0,o5
  ProcessTime : EventBasedRandomNumber  meanExp=0.05  minUnif=1  meanNorm=2  stdNorm=0.2  Seed=20443
  Routing : EventBasedRandomNumber  Distribution=Arbitrary discrete  valueVecDisc=[0,1,2,3,4,5,6,7,8,9,10,11,12,13,14,15,16,17,18,19,20,21,22,23,24,25,26,27,28,29,30,31,32,33,34,35,36,37,38,39,40,41,42,43,44,45,46,47]  probVecDisc=[0,0.0221,0.0037,0.0074,0.0294,0.0184,0.0221,0.011,0.0331,0.0331,0.0184,0.0184,0.0257,0.0361,0.0074,0.0331,0.011,0.0257,0.0074,0.0221,0.0221,0.011,0.0074,0.0037,0.0221,0.0221,0.0331,0.0184,0.0368,0.0257,0.0257,0.0184,0.0331,0.0074,0.0221,0.0331,0.0074,0.0184,0.0221,0.0331,0.0257,0.0331,0.0074,0.0221,0.0257,0.0331,0.0184,0.0257]  Seed=23660
  read_ProcessTimer : ReadTimer  TimerTag=T_Process_96  StatAverageTimeElapsed=on
      settings: OutputPortMap=o3
  setRouting : SetAttribute  AttributeName=outputFlowNode  AttributeFrom=Signal port  EvaluatedAttributeValue={ []}
  start_ProcessTimer : StartTimer  TimerTag=T_Process_96  TimerStartedOption=Restart
  IN_Job : PMIOPort  Port=1  Side=Left
  OUT_Job : PMIOPort  Port=2  Side=Right
  wires:
  Routing/1 -> setRouting/1
  ProcessTime/1 -> ProcessServer/1
  connections:
  setRouting/LConn1 -- OUTQueue/RConn1
  IN_Job/RConn1 -- start_ProcessTimer/LConn1
  ProcessServer/RConn1 -- read_ProcessTimer/LConn1
  start_ProcessTimer/RConn1 -- ProcessQueue/LConn1
  ProcessQueue/RConn1 -- ProcessServer/LConn1
  read_ProcessTimer/RConn1 -- OUTQueue/LConn1
  OUT_Job/RConn1 -- setRouting/RConn1

== system ProcessNetworkSimulation/Process_97/Process ==
  OUTQueue : FIFOQueue  Capacity=inf
  ProcessQueue : FIFOQueue  Capacity=Inf  StatAverageWait=on  StatAverageQueueLength=on
      settings: OutputPortMap=o2,o3
  ProcessServer : NServer  NumberOfServers=9  ServiceTimeFrom=Signal port t  StatNumberDeparted=on  StatUtilization=on
      settings: OutputPortMap=o0,o5
  ProcessTime : EventBasedRandomNumber  meanExp=0.05  minUnif=1  meanNorm=2  stdNorm=0.2  Seed=26877
  Routing : EventBasedRandomNumber  Distribution=Arbitrary discrete  valueVecDisc=[0,1,2,3,4,5,6,7,8,9,10,11,12,13,14,15,16,17,18,19,20,21,22,23,24,25,26,27,28,29,30]  probVecDisc=[0,0.0178,0.0355,0.0533,0.0296,0.0589,0.0533,0.0414,0.0059,0.0414,0.0533,0.0059,0.0533,0.0414,0.0296,0.0355,0.0533,0.0414,0.0059,0.0414,0.0178,0.0533,0.0533,0.0414,0.0118,0.0533,0.0118,0.0178,0.0118,0.0296,0]  Seed=30094
  read_ProcessTimer : ReadTimer  TimerTag=T_Process_97  StatAverageTimeElapsed=on
      settings: OutputPortMap=o3
  setRouting : SetAttribute  AttributeName=outputFlowNode  AttributeFrom=Signal port  EvaluatedAttributeValue={ []}
  start_ProcessTimer : StartTimer  TimerTag=T_Process_97  TimerStartedOption=Restart
  IN_Job : PMIOPort  Port=1  Side=Left
  OUT_Job : PMIOPort  Port=2  Side=Right
  wires:
  Routing/1 -> setRouting/1
  ProcessTime/1 -> ProcessServer/1
  connections:
  setRouting/LConn1 -- OUTQueue/RConn1
  IN_Job/RConn1 -- start_ProcessTimer/LConn1
  ProcessServer/RConn1 -- read_ProcessTimer/LConn1
  start_ProcessTimer/RConn1 -- ProcessQueue/LConn1
  ProcessQueue/RConn1 -- ProcessServer/LConn1
  read_ProcessTimer/RConn1 -- OUTQueue/LConn1
  OUT_Job/RConn1 -- setRouting/RConn1

== system ProcessNetworkSimulation/Process_98/Process ==
  OUTQueue : FIFOQueue  Capacity=inf
  ProcessQueue : FIFOQueue  Capacity=Inf  StatAverageWait=on  StatAverageQueueLength=on
      settings: OutputPortMap=o2,o3
  ProcessServer : NServer  NumberOfServers=12  ServiceTimeFrom=Signal port t  StatNumberDeparted=on  StatUtilization=on
      settings: OutputPortMap=o0,o5
  ProcessTime : EventBasedRandomNumber  meanExp=0.05  minUnif=1  meanNorm=2  stdNorm=0.2  Seed=33311
  Routing : EventBasedRandomNumber  Distribution=Arbitrary discrete  valueVecDisc=[0,1,2,3,4,5,6,7,8,9,10,11,12,13,14,15,16,17,18,19,20,21,22,23,24,25,26,27,28,29,30,31,32,33,34,35,36,37,38]  probVecDisc=[0,0.0281,0.0337,0.0112,0.0112,0.0281,0.0506,0.0112,0.0112,0.0112,0.0169,0.0169,0.0056,0.0337,0.0112,0.0337,0.0281,0.0337,0.0281,0.0112,0.0337,0.0112,0.0393,0.0506,0.0169,0.0112,0.0169,0.0506,0.0337,0.0281,0.0393,0.0169,0.0393,0.0281,0.0506,0.0393,0.0506,0.0281,0]  Seed=36528
  read_ProcessTimer : ReadTimer  TimerTag=T_Process_98  StatAverageTimeElapsed=on
      settings: OutputPortMap=o3
  setRouting : SetAttribute  AttributeName=outputFlowNode  AttributeFrom=Signal port  EvaluatedAttributeValue={ []}
  start_ProcessTimer : StartTimer  TimerTag=T_Process_98  TimerStartedOption=Restart
  IN_Job : PMIOPort  Port=1  Side=Left
  OUT_Job : PMIOPort  Port=2  Side=Right
  wires:
  Routing/1 -> setRouting/1
  ProcessTime/1 -> ProcessServer/1
  connections:
  setRouting/LConn1 -- OUTQueue/RConn1
  IN_Job/RConn1 -- start_ProcessTimer/LConn1
  ProcessServer/RConn1 -- read_ProcessTimer/LConn1
  start_ProcessTimer/RConn1 -- ProcessQueue/LConn1
  ProcessQueue/RConn1 -- ProcessServer/LConn1
  read_ProcessTimer/RConn1 -- OUTQueue/LConn1
  OUT_Job/RConn1 -- setRouting/RConn1
